simulink model "simulation_w_switch"  (Simulink 10.0)
settings: Solver=VariableStepAuto  StartTime=0.0  StopTime=tTot  MaxStep=1e-4  RelTol=1e-3
PreLoadFcn:
  | syst_init
values from neighbouring files (symbols this model uses):
  D = diag(Ir.^-1)    [syst_init.m]
  DGU = stateDyn(DGU,6)    [syst_init.m]
  Il_bar1 = 5/3    (= 1.66666666667)    [syst_init.m]
  Il_bar2 = 6/3    (= 2)    [syst_init.m]
  Il_bar3 = 7/3    (= 2.33333333333)    [syst_init.m]
  Il_bar4 = 6.5/3    (= 2.16666666667)    [syst_init.m]
  Il_bar5 = 8/3    (= 2.66666666667)    [syst_init.m]
  Il_bar6 = 7.5/3    (= 2.5)    [syst_init.m]
  L_first = Bc_first*Wcomm_first*(Bc_first')    [syst_init.m]
  L_full = Bc_full*Wcomm_full*(Bc_full')    [syst_init.m]
  L_unp = Bc_unp*Wcomm_unp*(Bc_unp')    [syst_init.m]
  N = 6    [syst_init.m]
  Pl_bar1 = 100/3    (= 33.3333333333)    [syst_init.m]
  Pl_bar2 = 120/3    (= 40)    [syst_init.m]
  Pl_bar3 = 105/3    (= 35)    [syst_init.m]
  Pl_bar4 = 95/3    (= 31.6666666667)    [syst_init.m]
  Pl_bar5 = 110/3    (= 36.6666666667)    [syst_init.m]
  Pl_bar6 = 105/3    (= 35)    [syst_init.m]
  T_zie_change = 17    [syst_init.m]
  T_zip_change = 6    [syst_init.m]
  Tc = 1.5    [syst_init.m]
  Tcommfail = tTot-3    (= 26)    [syst_init.m]
  Tplg = 10    [syst_init.m]
  Tunp = 22    [syst_init.m]
  Vref1 = 47    [syst_init.m]
  Vref2 = 48    [syst_init.m]
  Vref3 = 45    [syst_init.m]
  Vref4 = 50    [syst_init.m]
  Vref5 = 46    [syst_init.m]
  Vref6 = 49    [syst_init.m]
  Vs = 80    [syst_init.m]
  Yl_bar1 = 1/10/3    (= 0.0333333333333)    [syst_init.m]
  Yl_bar2 = 1/9/3    (= 0.037037037037)    [syst_init.m]
  Yl_bar3 = 1/11/3    (= 0.030303030303)    [syst_init.m]
  Yl_bar4 = 1/11/3    (= 0.030303030303)    [syst_init.m]
  Yl_bar5 = 1/10/3    (= 0.0333333333333)    [syst_init.m]
  Yl_bar6 = 1/10.5/3    (= 0.031746031746)    [syst_init.m]
undefined symbols (not defined in the file or in its folder): L
libraries: powerlib x135, powerlib_meascontrol x6
(part 1 of 2)
settings Model: Creator=mustafa  LastModifiedBy=mustafa
settings DataIOCC: SaveFormat=Dataset
settings OptimizationCC: LifeSpan=auto
settings DebuggingCC: UnderspecifiedInitializationDetection=Simplified  MergeDetectMultiDrivingBlocksExec=error  UnconnectedInputMsg=none  UnconnectedOutputMsg=none  UnconnectedLineMsg=none  SFUnexpectedBacktrackingDiag=error  SFNoUnconditionalDefaultTransitionDiag=error  SFExecutionAtInitializationDiag=warning
settings HardwareCC: ProdBitPerPointer=64  ProdBitPerSizeT=64  ProdBitPerPtrDiffT=64  ProdLargestAtomicFloat=Float  ProdIntDivRoundTo=Zero  ProdEndianess=LittleEndian  ProdWordSize=64  ProdHWDeviceType=Intel->x86-64 (Windows64)
settings ModelReferenceCC: PropagateSignalLabelsOutOfModel=on
settings SFSimCC: SimUseLocalCustomCode=on
settings RTWCC: RTWUseLocalCustomCode=on
settings CodeAppCC: StateflowObjectComments=off
settings GRTTargetCC: TargetLangStandard=C99 (ISO)  CombineOutputUpdateFcns=on  GRTInterface=off
settings ConfigComp: CovMetricSettings=dwe  CovHtmlReporting=off  CovSaveCumulativeToWorkspaceVar=off  CovSaveSingleToWorkspaceVar=off

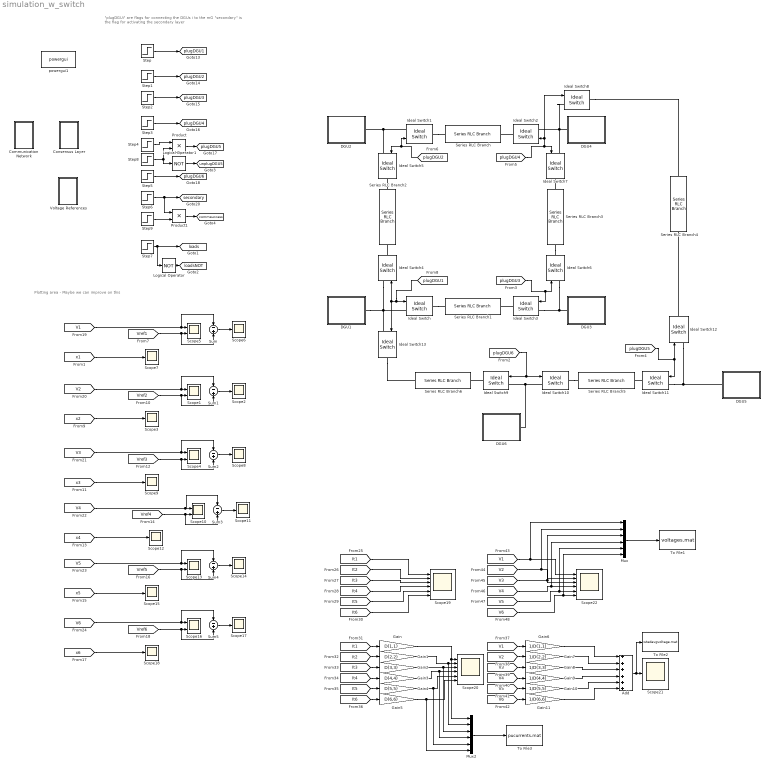
== system simulation_w_switch ==
  note: Plotting area - Maybe we can improve on this
  note: "plugDGUi" are flags for connecting the DGUs i to the mG
      | "secondary" is the flag for activating the secondary layer
  Add : Sum  Inputs=++++++
  Communication  Network : Subsystem
  Consensus Layer : Subsystem
  DGU1 : Subsystem
  DGU2 : Subsystem
  DGU3 : Subsystem
  DGU4 : Subsystem
  DGU5 : Subsystem
  DGU6 : Subsystem
  Gain : Gain  Gain=D(1,1)
  Gain1 : Gain  Gain=D(2,2)
  Gain10 : Gain  Gain=1/D(5,5)
  Gain11 : Gain  Gain=1/D(6,6)
  Gain2 : Gain  Gain=D(3,3)
  Gain3 : Gain  Gain=D(4,4)
  Gain4 : Gain  Gain=D(5,5)
  Gain5 : Gain  Gain=D(6,6)
  Gain6 : Gain  Gain=1/D(1,1)
  Gain7 : Gain  Gain=1/D(2,2)
  Gain8 : Gain  Gain=1/D(3,3)
  Gain9 : Gain  Gain=1/D(4,4)
  Ideal Switch{,1..13} (14 alike) : powerlib/Power Electronics/Ideal Switch  Ron=0.001  Lon=0  IC=0  Rs=1e5  Cs=inf  Measurements=off
      settings: SourceProductName=Simscape Electrical
  Logical Operator : Logic  Operator=NOT  AllPortsSameDT=off  OutDataTypeStr=boolean
  Logical Operator1 : Logic  Operator=NOT  AllPortsSameDT=off  OutDataTypeStr=boolean
  Mux : Mux  Inputs=6
  Mux2 : Mux  Inputs=6
  Product : Product
  Product1 : Product
  Scope{1,4..5,10,13,16} (6 alike) : Scope  NumInputPorts=2
  Scope{2..3,6..9,11..12,14..15,17..18,21} (13 alike) : Scope
  Scope19 : Scope  NumInputPorts=6
  Scope20 : Scope  NumInputPorts=6
  Scope22 : Scope  NumInputPorts=6
  Series RLC Branch : powerlib/Elements/Series RLC Branch  LConnTagsString=__new0  RConnTagsString=__new0  BranchType=RL  Resistance=DGU(2).Rij(2)  Inductance=DGU(2).Lij(2)  SetiL0=off  InitialCurrent=0  Capacitance=1e-6  Setx0=off  InitialVoltage=0  Measurements=None
      settings: SourceProductName=Simscape Electrical
  Series RLC Branch1 : powerlib/Elements/Series RLC Branch  LConnTagsString=__new0  RConnTagsString=__new0  BranchType=RL  Resistance=DGU(1).Rij(2)  Inductance=DGU(1).Lij(2)  SetiL0=off  InitialCurrent=0  Capacitance=1e-6  Setx0=off  InitialVoltage=0  Measurements=None
      settings: SourceProductName=Simscape Electrical
  Series RLC Branch2 : powerlib/Elements/Series RLC Branch  LConnTagsString=__new0  RConnTagsString=__new0  BranchType=RL  Resistance=DGU(1).Rij(1)  Inductance=DGU(1).Lij(1)  SetiL0=off  InitialCurrent=0  Capacitance=1e-6  Setx0=off  InitialVoltage=0  Measurements=None
      settings: SourceProductName=Simscape Electrical
  Series RLC Branch3 : powerlib/Elements/Series RLC Branch  LConnTagsString=__new0  RConnTagsString=__new0  BranchType=RL  Resistance=DGU(3).Rij(2)  Inductance=DGU(3).Lij(2)  SetiL0=off  InitialCurrent=0  Capacitance=1e-6  Setx0=off  InitialVoltage=0  Measurements=None
      settings: SourceProductName=Simscape Electrical
  Series RLC Branch4 : powerlib/Elements/Series RLC Branch  LConnTagsString=__new0  RConnTagsString=__new0  BranchType=RL  Resistance=DGU(4).Rij(3)  Inductance=DGU(4).Lij(3)  SetiL0=off  InitialCurrent=0  Capacitance=1e-6  Setx0=off  InitialVoltage=0  Measurements=None
      settings: SourceProductName=Simscape Electrical
  Series RLC Branch5 : powerlib/Elements/Series RLC Branch  LConnTagsString=__new0  RConnTagsString=__new0  BranchType=RL  Resistance=DGU(5).Rij(2)  Inductance=DGU(5).Lij(2)  SetiL0=off  InitialCurrent=0  Capacitance=1e-6  Setx0=off  InitialVoltage=0  Measurements=None
      settings: SourceProductName=Simscape Electrical
  Series RLC Branch6 : powerlib/Elements/Series RLC Branch  LConnTagsString=__new0  RConnTagsString=__new0  BranchType=RL  Resistance=DGU(1).Rij(3)  Inductance=DGU(1).Lij(3)  SetiL0=off  InitialCurrent=0  Capacitance=1e-6  Setx0=off  InitialVoltage=0  Measurements=None
      settings: SourceProductName=Simscape Electrical
  Step{,1..4,6} (6 alike) : Step  Time=Tc  SampleTime=0
  Step5 : Step  Time=Tplg  SampleTime=0
  Step7 : Step  Time=Tc-0.1  SampleTime=0
  Step8 : Step  Time=Tunp  Before=1  After=0  SampleTime=0
  Step9 : Step  Time=Tcommfail  Before=1  After=0  SampleTime=0
  Sum{,1..5} (6 alike) : Sum  Inputs=-|+
  To File1 : ToFile  Filename=voltages.mat  MatrixName=V  SaveFormat=Timeseries
  To File2 : ToFile  Filename=wtedavgvoltage.mat  MatrixName=Vavg  SaveFormat=Timeseries
  To File3 : ToFile  Filename=pucurrents.mat  MatrixName=Itpu  SaveFormat=Timeseries
  Voltage References : Subsystem
  powergui1 : powerlib/powergui  Priority=1  SimulationMode=Continuous  SampleTime=50e-6  frequency=60  Iterations=50  frequencyindice=0  Pbase=100e6  ErrMax=1e-4  UnitsV=kV  UnitsW=MW  buscounter=0  FunctionMessages=off  echomessages=off  EnableUseOfTLC=off  CurrentSourceSwitches=off  DisableSnubberDevices=off  DisableRonSwitches=off  DisableVfSwitches=off  DisplayEquations=off  AutomaticDiscreteSolvers=off  SolverType=Tustin/Backward Euler (TBE)  Interpol=off  ExternalGateDelay=off  methode=off  Ts=100  x0status=blocks  SPID=on  SwTol=0  HookPort=off  NonlinearTolerance=1e-4  nMaxIteration=100  ContinueOnMaxIteration=off  RestoreLinks=warning  ResistiveCurrentMeasurement=off  Frange=[0:2:500]  Ylog=off  Xlog=on  ShowGrid=off  save=off  variable=ZData  structure=0  ZoomFFT=off  StartTime=0.0  cycles=1  DisplayStyle=1  fundamental=60  FreqAxis=off  MaxFrequency=1000  frequencyindicesteady=1  RmsSteady=1  display=off
      settings: SourceProductName=Simscape Electrical
  tag scope: commsuccess=global, loads=global, loadsNOT=global, plugDGU1=global, plugDGU2=global, plugDGU3=global, plugDGU4=global, plugDGU5=global, plugDGU6=global, secondary=global, unplugDGU5=global
  wires:
  [Vref1] -> Sum/2, Scope5/2
  [V1] -> Sum/1, Scope5/1
  Sum/1 -> Scope6/1
  [x1] -> Scope7/1
  [plugDGU2] -> Ideal Switch1/1, Ideal Switch5/1
  [plugDGU1] -> Ideal Switch4/1, Ideal Switch13/1, Ideal Switch/1
  [plugDGU3] -> Ideal Switch6/1, Ideal Switch3/1
  [plugDGU4] -> Ideal Switch7/1, Ideal Switch8/1, Ideal Switch2/1
  [plugDGU6] -> Ideal Switch9/1, Ideal Switch10/1
  [plugDGU5] -> Ideal Switch11/1, Ideal Switch12/1
  [V2] -> Sum1/1, Scope1/1
  [Vref2] -> Sum1/2, Scope1/2
  Sum1/1 -> Scope2/1
  [x2] -> Scope3/1
  [V3] -> Sum2/1, Scope4/1
  [Vref3] -> Sum2/2, Scope4/2
  Sum2/1 -> Scope8/1
  [x3] -> Scope9/1
  [V4] -> Sum3/1, Scope10/1
  [Vref4] -> Sum3/2, Scope10/2
  Sum3/1 -> Scope11/1
  [x4] -> Scope12/1
  [V5] -> Sum4/1, Scope13/1
  [Vref5] -> Sum4/2, Scope13/2
  Sum4/1 -> Scope14/1
  [x5] -> Scope15/1
  [V6] -> Sum5/1, Scope16/1
  [Vref6] -> Sum5/2, Scope16/2
  Sum5/1 -> Scope17/1
  [x6] -> Scope18/1
  Step/1 -> [plugDGU1]
  Step1/1 -> [plugDGU2]
  Step2/1 -> [plugDGU3]
  Step3/1 -> [plugDGU4]
  Step5/1 -> [plugDGU6]
  Step6/1 -> Product1/1, [secondary]
  [It3] -> Scope19/3
  [It2] -> Scope19/2
  [It1] -> Scope19/1
  [It4] -> Scope19/4
  [It5] -> Scope19/5
  [It6] -> Scope19/6
  [V6] -> Mux/6, Scope22/6
  [V1] -> Mux/1, Scope22/1
  [V4] -> Mux/4, Scope22/4
  [V3] -> Mux/3, Scope22/3
  [V2] -> Mux/2, Scope22/2
  [V5] -> Mux/5, Scope22/5
  Step7/1 -> Logical Operator/1, [loads]
  Logical Operator/1 -> [loadsNOT]
  Product/1 -> [plugDGU5]
  Step4/1 -> Product/1
  Step8/1 -> Logical Operator1/1, Product/2
  Logical Operator1/1 -> [unplugDGU5]
  [It1] -> Gain/1
  [It2] -> Gain1/1
  [It3] -> Gain2/1
  [It4] -> Gain3/1
  [It5] -> Gain4/1
  [It6] -> Gain5/1
  Gain5/1 -> Mux2/6, Scope20/6
  Gain4/1 -> Mux2/5, Scope20/5
  Gain3/1 -> Mux2/4, Scope20/4
  Gain2/1 -> Scope20/3, Mux2/3
  Gain1/1 -> Mux2/2, Scope20/2
  Gain/1 -> Mux2/1, Scope20/1
  Step9/1 -> Product1/2
  Product1/1 -> [commsuccess]
  Gain6/1 -> Add/1
  Gain7/1 -> Add/2
  Gain8/1 -> Add/3
  Gain9/1 -> Add/4
  Gain10/1 -> Add/5
  Gain11/1 -> Add/6
  [V6] -> Gain11/1
  [V5] -> Gain10/1
  [V4] -> Gain9/1
  [V3] -> Gain8/1
  [V2] -> Gain7/1
  [V1] -> Gain6/1
  Mux/1 -> To File1/1
  Mux2/1 -> To File3/1
  Add/1 -> To File2/1, Scope21/1
  connections:
  Ideal Switch/RConn1 -- Series RLC Branch1/LConn1
  Ideal Switch1/RConn1 -- Series RLC Branch/LConn1
  Ideal Switch4/RConn1 -- Series RLC Branch2/RConn1
  DGU1/RConn1 -- Ideal Switch13/LConn1 -- Ideal Switch4/LConn1 -- Ideal Switch/LConn1
  Ideal Switch5/RConn1 -- Series RLC Branch2/LConn1
  Ideal Switch1/LConn1 -- Ideal Switch5/LConn1 -- DGU2/RConn1
  Ideal Switch3/RConn1 -- Series RLC Branch1/RConn1
  Ideal Switch2/RConn1 -- Series RLC Branch/RConn1
  Ideal Switch3/LConn1 -- Ideal Switch6/LConn1 -- DGU3/LConn1
  Ideal Switch2/LConn1 -- Ideal Switch8/LConn1 -- Ideal Switch7/LConn1 -- DGU4/LConn1
  Series RLC Branch3/LConn1 -- Ideal Switch7/RConn1
  Series RLC Branch3/RConn1 -- Ideal Switch6/RConn1
  Ideal Switch8/RConn1 -- Series RLC Branch4/LConn1
  Ideal Switch9/RConn1 -- Series RLC Branch6/RConn1
  Ideal Switch10/RConn1 -- Series RLC Branch5/LConn1
  Ideal Switch10/LConn1 -- Ideal Switch9/LConn1 -- DGU6/RConn1
  Ideal Switch11/RConn1 -- Series RLC Branch5/RConn1
  Ideal Switch11/LConn1 -- Ideal Switch12/LConn1 -- DGU5/LConn1
  Ideal Switch13/RConn1 -- Series RLC Branch6/LConn1
  Ideal Switch12/RConn1 -- Series RLC Branch4/RConn1

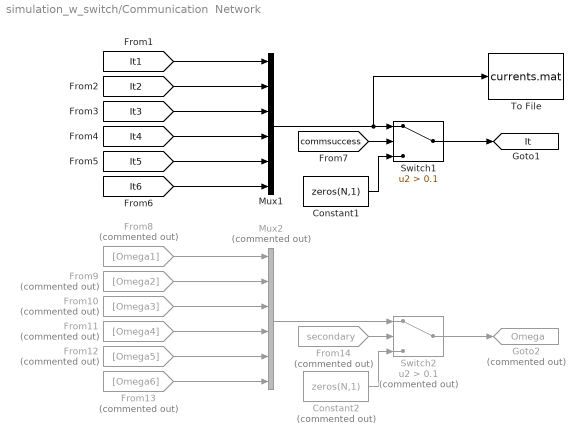
== system simulation_w_switch/Communication  Network ==
  Constant1 : Constant  Value=zeros(N,1)
  Constant2 : Constant  Commented=on  Value=zeros(N,1)
  From10 : From  Commented=on  GotoTag=Omega3  TagVisibility=global
  From11 : From  Commented=on  GotoTag=Omega4  TagVisibility=global
  From12 : From  Commented=on  GotoTag=Omega5  TagVisibility=global
  From13 : From  Commented=on  GotoTag=Omega6  TagVisibility=global
  From14 : From  Commented=on  GotoTag=secondary  TagVisibility=global
  From8 : From  Commented=on  GotoTag=Omega1  TagVisibility=global
  From9 : From  Commented=on  GotoTag=Omega2  TagVisibility=global
  Goto2 : Goto  Commented=on  GotoTag=Omega  TagVisibility=global
  Mux1 : Mux  Inputs=6
  Mux2 : Mux  Commented=on  Inputs=6
  Switch1 : Switch  Criteria=u2 > Threshold  Threshold=0.1
  Switch2 : Switch  Commented=on  Criteria=u2 > Threshold  Threshold=0.1
  To File : ToFile  Filename=currents.mat  MatrixName=It  SaveFormat=Timeseries
  tag scope: It=global
  wires:
  Mux1/1 -> To File/1, Switch1/1
  Switch1/1 -> [It]
  [commsuccess] -> Switch1/2
  Constant1/1 -> Switch1/3
  [It2] -> Mux1/2
  [It3] -> Mux1/3
  [It4] -> Mux1/4
  [It5] -> Mux1/5
  [It6] -> Mux1/6
  [It1] -> Mux1/1
  From8/1 -> Mux2/1
  From13/1 -> Mux2/6
  From12/1 -> Mux2/5
  From11/1 -> Mux2/4
  From10/1 -> Mux2/3
  From9/1 -> Mux2/2
  Constant2/1 -> Switch2/3
  From14/1 -> Switch2/2
  Switch2/1 -> Goto2/1
  Mux2/1 -> Switch2/1

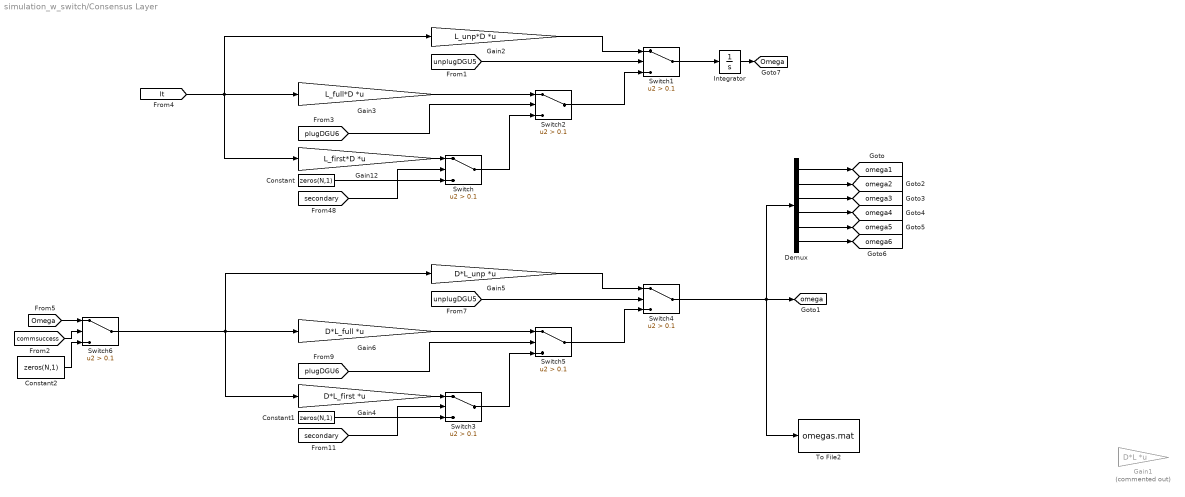
== system simulation_w_switch/Consensus Layer ==
  Constant : Constant  Value=zeros(N,1)
  Constant1 : Constant  Value=zeros(N,1)
  Constant2 : Constant  Value=zeros(N,1)
  Demux : Demux  Outputs=6
  Gain1 : Gain  Commented=on  Gain=D*L  Multiplication=Matrix(K*u) (u vector)
  Gain12 : Gain  Gain=L_first*D  Multiplication=Matrix(K*u) (u vector)
  Gain2 : Gain  Gain=L_unp*D  Multiplication=Matrix(K*u) (u vector)
  Gain3 : Gain  Gain=L_full*D  Multiplication=Matrix(K*u) (u vector)
  Gain4 : Gain  Gain=D*L_first  Multiplication=Matrix(K*u) (u vector)
  Gain5 : Gain  Gain=D*L_unp  Multiplication=Matrix(K*u) (u vector)
  Gain6 : Gain  Gain=D*L_full  Multiplication=Matrix(K*u) (u vector)
  Integrator : Integrator
  Switch{,1..6} (7 alike) : Switch  Criteria=u2 > Threshold  Threshold=0.1
  To File2 : ToFile  Filename=omegas.mat  MatrixName=omega  SaveFormat=Timeseries
  tag scope: Omega=global, omega1=global, omega2=global, omega3=global, omega4=global, omega5=global, omega6=global, omega=global
  wires:
  Constant/1 -> Switch/3
  [secondary] -> Switch/2
  Switch4/1 -> To File2/1, Demux/1, [omega]
  Gain12/1 -> Switch/1
  Demux/1 -> [omega1]
  Demux/6 -> [omega6]
  Demux/5 -> [omega5]
  Demux/4 -> [omega4]
  Demux/3 -> [omega3]
  Demux/2 -> [omega2]
  Switch1/1 -> Integrator/1
  Switch2/1 -> Switch1/3
  [unplugDGU5] -> Switch1/2
  Gain2/1 -> Switch1/1
  [It] -> Gain12/1, Gain2/1, Gain3/1
  Switch/1 -> Switch2/3
  [plugDGU6] -> Switch2/2
  Gain3/1 -> Switch2/1
  Integrator/1 -> [Omega]
  Gain6/1 -> Switch5/1
  [plugDGU6] -> Switch5/2
  Switch3/1 -> Switch5/3
  Gain5/1 -> Switch4/1
  [unplugDGU5] -> Switch4/2
  Switch5/1 -> Switch4/3
  Gain4/1 -> Switch3/1
  [secondary] -> Switch3/2
  Constant1/1 -> Switch3/3
  Switch6/1 -> Gain4/1, Gain6/1, Gain5/1
  Constant2/1 -> Switch6/3
  [commsuccess] -> Switch6/2
  [Omega] -> Switch6/1

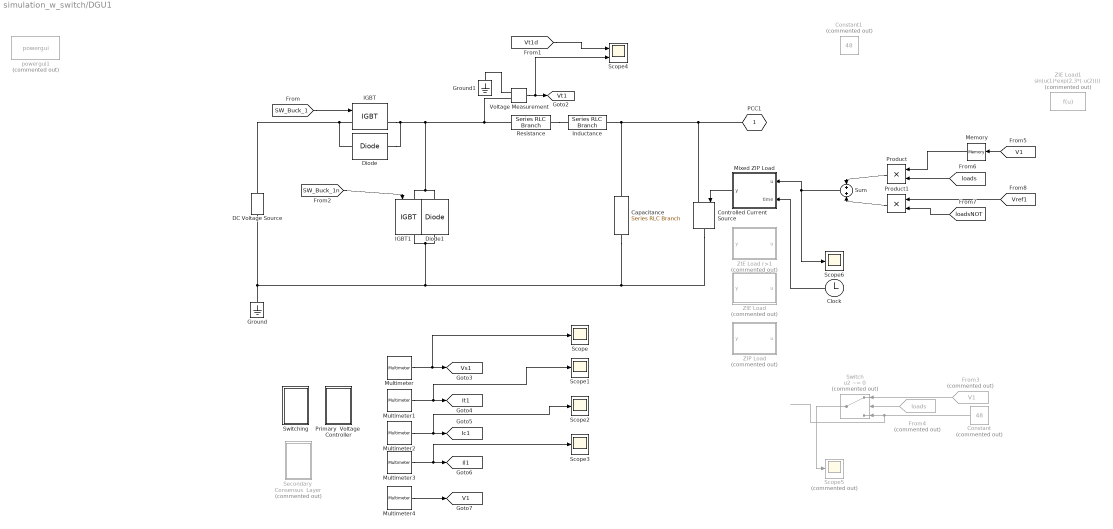
== system simulation_w_switch/DGU1 ==
  Capacitance : powerlib/Elements/Series RLC Branch  LConnTagsString=__new0  RConnTagsString=__new0  BranchType=C  Resistance=1  Inductance=1.8e-3  SetiL0=off  InitialCurrent=0  Capacitance=DGU(1).Ct  Setx0=on  InitialVoltage=48  Measurements=Branch voltage and current
      settings: SourceProductName=Simscape Electrical
  Clock : Clock
  Constant : Constant  Commented=on  Value=48
  Constant1 : Constant  Commented=on  Value=48
  Controlled Current Source : powerlib/Electrical Sources/Controlled Current Source  Initialize=on  Source_Type=DC  Amplitude=Il_bar1  Phase=0  Frequency=0  Measurements=Current
      settings: SourceProductName=Simscape Electrical
  DC Voltage Source : powerlib/Electrical Sources/DC Voltage Source  Amplitude=Vs  Measurements=Voltage
      settings: SourceProductName=Simscape Electrical
  Diode : powerlib/Power Electronics/Diode  Ron=0.001  Lon=0  Vf=0.8  IC=0  UseSnubber=0  Rs=500  Cs=250e-9  Measurements=off
      settings: SourceProductName=Simscape Electrical
  Diode1 : powerlib/Power Electronics/Diode  Ron=0.001  Lon=0  Vf=0.8  IC=0  UseSnubber=0  Rs=500  Cs=250e-9  Measurements=off
      settings: SourceProductName=Simscape Electrical
  From3 : From  Commented=on  GotoTag=V1  TagVisibility=global
  From4 : From  Commented=on  GotoTag=loads  TagVisibility=global
  Ground : powerlib/Elements/Ground  LConnTagsString=a
      settings: SourceProductName=Simscape Electrical
  Ground1 : powerlib/Elements/Ground  LConnTagsString=a
      settings: SourceProductName=Simscape Electrical
  IGBT : powerlib/Power Electronics/IGBT  Ron=0.001  Lon=0  Vf=1  Tf=1e-6  Tt=2e-6  IC=0  Rs=1e5  Cs=inf  Measurements=on
      settings: SourceProductName=Simscape Electrical
  IGBT1 : powerlib/Power Electronics/IGBT  Ron=0.001  Lon=0  Vf=1  Tf=1e-6  Tt=2e-6  IC=0  Rs=1e5  Cs=inf  Measurements=on
      settings: SourceProductName=Simscape Electrical
  Inductance : powerlib/Elements/Series RLC Branch  LConnTagsString=__new0  RConnTagsString=__new0  BranchType=L  Resistance=1  Inductance=DGU(1).Lt  SetiL0=on  InitialCurrent=Il_bar1  Capacitance=1e-6  Setx0=off  InitialVoltage=0  Measurements=None
      settings: SourceProductName=Simscape Electrical
  Memory : Memory
  Mixed ZIP Load : MATLAB Function  TreatAsAtomicUnit=on
  Multimeter : powerlib/Measurements/Multimeter  PhasorSimulation=off  OutputType=Complex  sel=7  L=30  Gain=1  yselected={'Usrc: DGU1/DC Voltage Source'};  PSBOutputType=1  PSBequivalent=0  AxesSetting=[0,0.1,-100,100]  Display=0  SavedBlockNames=-11
      settings: SourceProductName=Simscape Electrical
  Multimeter1 : powerlib/Measurements/Multimeter  PhasorSimulation=off  OutputType=Complex  sel=14  L=30  Gain=1  yselected={'Ib: DGU1/Resistance'};  PSBOutputType=1  PSBequivalent=0  AxesSetting=[0,0.1,-100,100]  Display=0  SavedBlockNames=-11
      settings: SourceProductName=Simscape Electrical
  Multimeter2 : powerlib/Measurements/Multimeter  PhasorSimulation=off  OutputType=Complex  sel=13  L=30  Gain=1  yselected={'Ib: DGU1/Capacitance'};  PSBOutputType=1  PSBequivalent=0  AxesSetting=[0,0.1,-100,100]  Display=0  SavedBlockNames=-11
      settings: SourceProductName=Simscape Electrical
  Multimeter3 : powerlib/Measurements/Multimeter  PhasorSimulation=off  OutputType=Complex  sel=25  L=30  Gain=1  yselected={'Isrc: DGU1/Controlled Current Source'};  PSBOutputType=1  PSBequivalent=0  AxesSetting=[0,0.1,-100,100]  Display=0  SavedBlockNames=-11
      settings: SourceProductName=Simscape Electrical
  Multimeter4 : powerlib/Measurements/Multimeter  PhasorSimulation=off  OutputType=Complex  sel=1  L=30  Gain=1  yselected={'Ub: DGU1/Capacitance'};  PSBOutputType=1  PSBequivalent=0  AxesSetting=[0,0.1,-100,100]  Display=0  SavedBlockNames=-11
      settings: SourceProductName=Simscape Electrical
  Primary  Voltage  Controller : Subsystem
  Product : Product
  Product1 : Product
  Resistance : powerlib/Elements/Series RLC Branch  LConnTagsString=__new0  RConnTagsString=__new0  BranchType=R  Resistance=DGU(1).Rt  Inductance=1e-3  SetiL0=off  InitialCurrent=0  Capacitance=1e-6  Setx0=off  InitialVoltage=0  Measurements=Branch current
      settings: SourceProductName=Simscape Electrical
  Scope{,1..3,6} (5 alike) : Scope
  Scope4 : Scope  NumInputPorts=2
  Scope5 : Scope  Commented=on
  Secondary  Consensus  Layer : Subsystem  Commented=on
  Sum : Sum  Inputs=+|+
  Switch : Switch  Commented=on  Criteria=u2 ~= 0  Threshold=0.1
  Switching : Subsystem
  Voltage Measurement : powerlib/Measurements/Voltage Measurement  PhasorSimulation=off  OutputType=Complex  PSBequivalent=0
      settings: SourceProductName=Simscape Electrical
  ZIE Load : MATLAB Function  Commented=on  TreatAsAtomicUnit=on
  ZIE Load r>1 : MATLAB Function  Commented=on  TreatAsAtomicUnit=on
  ZIE Load1 : Fcn  Commented=on  Expr=sin(u(1)*exp(2.3*(-u(2))))
  ZIP Load : MATLAB Function  Commented=on  TreatAsAtomicUnit=on
  powergui1 : powerlib/powergui  Priority=1  Commented=on  SimulationMode=Continuous  SampleTime=50e-6  frequency=60  Iterations=50  frequencyindice=60  Pbase=100e6  ErrMax=1e-4  UnitsV=kV  UnitsW=MW  buscounter=0  FunctionMessages=off  echomessages=off  EnableUseOfTLC=off  CurrentSourceSwitches=off  DisableSnubberDevices=off  DisableRonSwitches=off  DisableVfSwitches=off  DisplayEquations=off  AutomaticDiscreteSolvers=off  SolverType=Tustin/Backward Euler (TBE)  Interpol=off  ExternalGateDelay=off  methode=off  Ts=100  x0status=blocks  SPID=on  SwTol=0  HookPort=off  NonlinearTolerance=1e-4  nMaxIteration=100  ContinueOnMaxIteration=off  RestoreLinks=warning  ResistiveCurrentMeasurement=off  Frange=[0:2:500]  Ylog=off  Xlog=on  ShowGrid=off  save=off  variable=ZData  structure=0  ZoomFFT=off  StartTime=0.0  cycles=1  DisplayStyle=1  fundamental=60  FreqAxis=off  MaxFrequency=1000  frequencyindicesteady=1  RmsSteady=1  display=off
      settings: SourceProductName=Simscape Electrical
  PCC1 : PMIOPort  Tag=PMCPort  Side=Right
  tag scope: Ic1=global, Il1=global, It1=global, V1=global, Vs1=global, Vt1=global
  wires:
  Multimeter/1 -> Scope/1, [Vs1]
  Multimeter2/1 -> Scope2/1, [Ic1]
  Voltage Measurement/1 -> Scope4/2, [Vt1]
  Multimeter1/1 -> Scope1/1, [It1]
  [SW_Buck_1n] -> IGBT1/1
  Multimeter3/1 -> Scope3/1, [Il1]
  [SW_Buck_1] -> IGBT/1
  Multimeter4/1 -> [V1]
  [Vt1d] -> Scope4/1
  Mixed ZIP Load/1(y) -> Controlled Current Source/1
  From4/1 -> Switch/2
  From3/1 -> Switch/1
  Constant/1 -> Switch/3
  Switch/1 -> Scope5/1
  [loads] -> Product/2
  [Vref1] -> Product1/1
  [loadsNOT] -> Product1/2
  Product/1 -> Sum/1
  Product1/1 -> Sum/2
  Sum/1 -> Mixed ZIP Load/1(u), Scope6/1
  [V1] -> Memory/1
  Memory/1 -> Product/1
  Clock/1 -> Mixed ZIP Load/2(time)
  connections:
  Ground1/LConn1 -- Voltage Measurement/LConn2
  IGBT1/RConn1 -- Controlled Current Source/RConn1 -- Capacitance/RConn1 -- Ground/LConn1 -- DC Voltage Source/LConn1 -- Diode1/LConn1
  Capacitance/LConn1 -- Controlled Current Source/LConn1 -- PCC1/RConn1 -- Inductance/RConn1
  IGBT1/LConn1 -- Resistance/LConn1 -- Voltage Measurement/LConn1 -- IGBT/RConn1 -- Diode/LConn1 -- Diode1/RConn1
  IGBT/LConn1 -- Diode/RConn1 -- DC Voltage Source/RConn1
  Resistance/RConn1 -- Inductance/LConn1

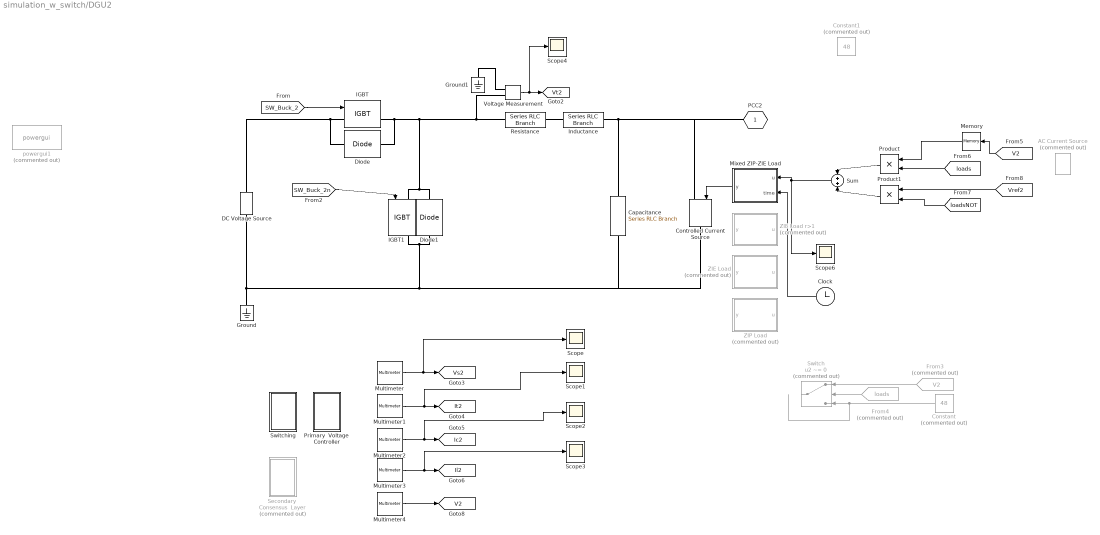
== system simulation_w_switch/DGU2 ==
  AC Current Source : powerlib/Electrical Sources/AC Current Source  Commented=on  Amplitude=12  Phase=90  Frequency=0  SampleTime=0  Measurements=Current
      settings: SourceProductName=Simscape Electrical  SourceProductBaseCode=PS
  Capacitance : powerlib/Elements/Series RLC Branch  LConnTagsString=__new0  RConnTagsString=__new0  BranchType=C  Resistance=1  Inductance=1.8e-3  SetiL0=off  InitialCurrent=0  Capacitance=DGU(2).Ct  Setx0=on  InitialVoltage=48  Measurements=Branch voltage and current
      settings: SourceProductName=Simscape Electrical
  Clock : Clock
  Constant : Constant  Commented=on  Value=48
  Constant1 : Constant  Commented=on  Value=48
  Controlled Current Source : powerlib/Electrical Sources/Controlled Current Source  Initialize=on  Source_Type=DC  Amplitude=Il_bar2  Phase=0  Frequency=0  Measurements=Current
      settings: SourceProductName=Simscape Electrical
  DC Voltage Source : powerlib/Electrical Sources/DC Voltage Source  Amplitude=Vs  Measurements=Voltage
      settings: SourceProductName=Simscape Electrical
  Diode : powerlib/Power Electronics/Diode  Ron=0.001  Lon=0  Vf=0.8  IC=0  UseSnubber=0  Rs=500  Cs=250e-9  Measurements=off
      settings: SourceProductName=Simscape Electrical
  Diode1 : powerlib/Power Electronics/Diode  Ron=0.001  Lon=0  Vf=0.8  IC=0  UseSnubber=0  Rs=500  Cs=250e-9  Measurements=off
      settings: SourceProductName=Simscape Electrical
  From3 : From  Commented=on  GotoTag=V2  TagVisibility=global
  From4 : From  Commented=on  GotoTag=loads  TagVisibility=global
  Ground : powerlib/Elements/Ground  LConnTagsString=a
      settings: SourceProductName=Simscape Electrical
  Ground1 : powerlib/Elements/Ground  LConnTagsString=a
      settings: SourceProductName=Simscape Electrical
  IGBT : powerlib/Power Electronics/IGBT  Ron=0.001  Lon=0  Vf=1  Tf=1e-6  Tt=2e-6  IC=0  Rs=1e5  Cs=inf  Measurements=on
      settings: SourceProductName=Simscape Electrical
  IGBT1 : powerlib/Power Electronics/IGBT  Ron=0.001  Lon=0  Vf=1  Tf=1e-6  Tt=2e-6  IC=0  Rs=1e5  Cs=inf  Measurements=on
      settings: SourceProductName=Simscape Electrical
  Inductance : powerlib/Elements/Series RLC Branch  LConnTagsString=__new0  RConnTagsString=__new0  BranchType=L  Resistance=1  Inductance=DGU(2).Lt  SetiL0=on  InitialCurrent=Il_bar2  Capacitance=1e-6  Setx0=off  InitialVoltage=0  Measurements=None
      settings: SourceProductName=Simscape Electrical
  Memory : Memory
  Mixed ZIP-ZIE Load : MATLAB Function  TreatAsAtomicUnit=on
  Multimeter : powerlib/Measurements/Multimeter  PhasorSimulation=off  OutputType=Complex  sel=8  L=30  Gain=1  yselected={'Usrc: DGU2/DC Voltage Source'};  PSBOutputType=1  PSBequivalent=0  AxesSetting=[0,0.1,-100,100]  Display=0  SavedBlockNames=-11
      settings: SourceProductName=Simscape Electrical
  Multimeter1 : powerlib/Measurements/Multimeter  PhasorSimulation=off  OutputType=Complex  sel=16  L=30  Gain=1  yselected={'Ib: DGU2/Resistance'};  PSBOutputType=1  PSBequivalent=0  AxesSetting=[0,0.1,-100,100]  Display=0  SavedBlockNames=-11
      settings: SourceProductName=Simscape Electrical
  Multimeter2 : powerlib/Measurements/Multimeter  PhasorSimulation=off  OutputType=Complex  sel=15  L=30  Gain=1  yselected={'Ib: DGU2/Capacitance'};  PSBOutputType=1  PSBequivalent=0  AxesSetting=[0,0.1,-100,100]  Display=0  SavedBlockNames=-11
      settings: SourceProductName=Simscape Electrical
  Multimeter3 : powerlib/Measurements/Multimeter  PhasorSimulation=off  OutputType=Complex  sel=26  L=30  Gain=1  yselected={'Isrc: DGU2/Controlled Current Source'};  PSBOutputType=1  PSBequivalent=0  AxesSetting=[0,0.1,-100,100]  Display=0  SavedBlockNames=-11
      settings: SourceProductName=Simscape Electrical
  Multimeter4 : powerlib/Measurements/Multimeter  PhasorSimulation=off  OutputType=Complex  sel=2  L=30  Gain=1  yselected={'Ub: DGU2/Capacitance'};  PSBOutputType=1  PSBequivalent=0  AxesSetting=[0,0.1,-100,100]  Display=0  SavedBlockNames=-11
      settings: SourceProductName=Simscape Electrical
  Primary  Voltage  Controller : Subsystem
  Product : Product
  Product1 : Product
  Resistance : powerlib/Elements/Series RLC Branch  LConnTagsString=__new0  RConnTagsString=__new0  BranchType=R  Resistance=DGU(2).Rt  Inductance=1e-3  SetiL0=off  InitialCurrent=0  Capacitance=1e-6  Setx0=off  InitialVoltage=0  Measurements=Branch current
      settings: SourceProductName=Simscape Electrical
  Scope{,1..4,6} (6 alike) : Scope
  Secondary  Consensus  Layer : Subsystem  Commented=on
  Sum : Sum  Inputs=+|+
  Switch : Switch  Commented=on  Criteria=u2 ~= 0  Threshold=0.1
  Switching : Subsystem
  Voltage Measurement : powerlib/Measurements/Voltage Measurement  PhasorSimulation=off  OutputType=Complex  PSBequivalent=0
      settings: SourceProductName=Simscape Electrical
  ZIE Load : MATLAB Function  Commented=on  TreatAsAtomicUnit=on
  ZIE Load r>1 : MATLAB Function  Commented=on  TreatAsAtomicUnit=on
  ZIP Load : MATLAB Function  Commented=on  TreatAsAtomicUnit=on
  powergui1 : powerlib/powergui  Priority=1  Commented=on  SimulationMode=Continuous  SampleTime=50e-6  frequency=60  Iterations=50  frequencyindice=60  Pbase=100e6  ErrMax=1e-4  UnitsV=kV  UnitsW=MW  buscounter=0  FunctionMessages=off  echomessages=off  EnableUseOfTLC=off  CurrentSourceSwitches=off  DisableSnubberDevices=off  DisableRonSwitches=off  DisableVfSwitches=off  DisplayEquations=off  AutomaticDiscreteSolvers=off  SolverType=Tustin/Backward Euler (TBE)  Interpol=off  ExternalGateDelay=off  methode=off  Ts=100  x0status=blocks  SPID=on  SwTol=0  HookPort=off  NonlinearTolerance=1e-4  nMaxIteration=100  ContinueOnMaxIteration=off  RestoreLinks=warning  ResistiveCurrentMeasurement=off  Frange=[0:2:500]  Ylog=off  Xlog=on  ShowGrid=off  save=off  variable=ZData  structure=0  ZoomFFT=off  StartTime=0.0  cycles=1  DisplayStyle=1  fundamental=60  FreqAxis=off  MaxFrequency=1000  frequencyindicesteady=1  RmsSteady=1  display=off
      settings: SourceProductName=Simscape Electrical
  PCC2 : PMIOPort  Tag=PMCPort  Side=Right
  tag scope: Ic2=global, Il2=global, It2=global, V2=global, Vs2=global, Vt2=global
  wires:
  Multimeter/1 -> Scope/1, [Vs2]
  Multimeter2/1 -> Scope2/1, [Ic2]
  Voltage Measurement/1 -> Scope4/1, [Vt2]
  Multimeter1/1 -> Scope1/1, [It2]
  [SW_Buck_2n] -> IGBT1/1
  Multimeter3/1 -> Scope3/1, [Il2]
  [SW_Buck_2] -> IGBT/1
  Multimeter4/1 -> [V2]
  Mixed ZIP-ZIE Load/1(y) -> Controlled Current Source/1
  From4/1 -> Switch/2
  From3/1 -> Switch/1
  Constant/1 -> Switch/3
  [Vref2] -> Product1/1
  Product1/1 -> Sum/2
  Sum/1 -> Mixed ZIP-ZIE Load/1(u), Scope6/1
  [loadsNOT] -> Product1/2
  [loads] -> Product/2
  Memory/1 -> Product/1
  Product/1 -> Sum/1
  [V2] -> Memory/1
  Clock/1 -> Mixed ZIP-ZIE Load/2(time)
  connections:
  Ground1/LConn1 -- Voltage Measurement/LConn2
  IGBT1/RConn1 -- Controlled Current Source/RConn1 -- Capacitance/RConn1 -- Ground/LConn1 -- DC Voltage Source/LConn1 -- Diode1/LConn1
  Diode/LConn1 -- IGBT/RConn1 -- Resistance/LConn1 -- Voltage Measurement/LConn1 -- IGBT1/LConn1 -- Diode1/RConn1
  IGBT/LConn1 -- Diode/RConn1 -- DC Voltage Source/RConn1
  Resistance/RConn1 -- Inductance/LConn1
  Capacitance/LConn1 -- PCC2/RConn1 -- Controlled Current Source/LConn1 -- Inductance/RConn1

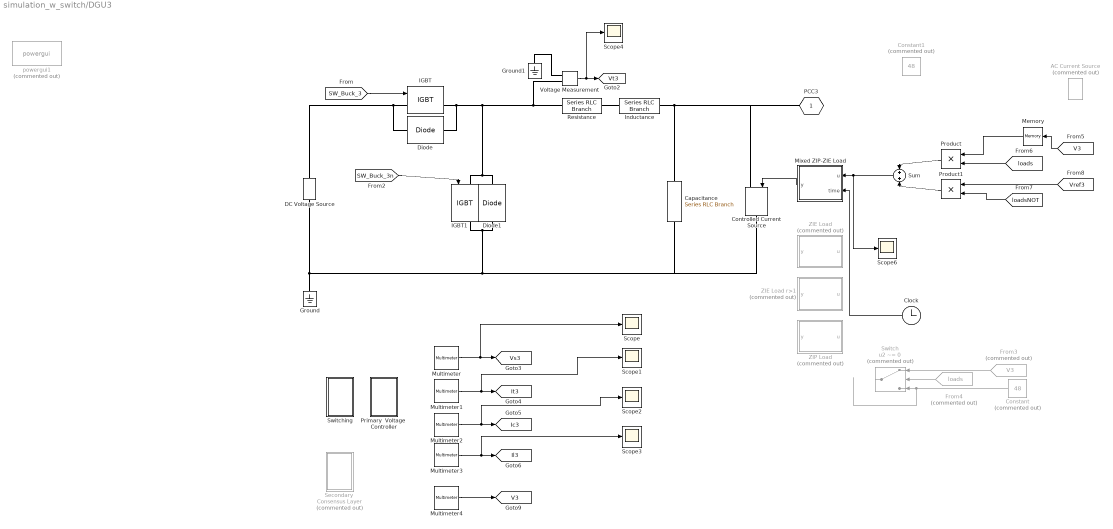
== system simulation_w_switch/DGU3 ==
  AC Current Source : powerlib/Electrical Sources/AC Current Source  Commented=on  Amplitude=15  Phase=90  Frequency=0  SampleTime=0  Measurements=Current
      settings: SourceProductName=Simscape Electrical  SourceProductBaseCode=PS
  Capacitance : powerlib/Elements/Series RLC Branch  LConnTagsString=__new0  RConnTagsString=__new0  BranchType=C  Resistance=1  Inductance=1.8e-3  SetiL0=off  InitialCurrent=0  Capacitance=DGU(3).Ct  Setx0=on  InitialVoltage=48  Measurements=Branch voltage and current
      settings: SourceProductName=Simscape Electrical
  Clock : Clock
  Constant : Constant  Commented=on  Value=48
  Constant1 : Constant  Commented=on  Value=48
  Controlled Current Source : powerlib/Electrical Sources/Controlled Current Source  Initialize=on  Source_Type=DC  Amplitude=Il_bar3  Phase=0  Frequency=0  Measurements=Current
      settings: SourceProductName=Simscape Electrical
  DC Voltage Source : powerlib/Electrical Sources/DC Voltage Source  Amplitude=Vs  Measurements=Voltage
      settings: SourceProductName=Simscape Electrical
  Diode : powerlib/Power Electronics/Diode  Ron=0.001  Lon=0  Vf=0.8  IC=0  UseSnubber=0  Rs=500  Cs=250e-9  Measurements=off
      settings: SourceProductName=Simscape Electrical
  Diode1 : powerlib/Power Electronics/Diode  Ron=0.001  Lon=0  Vf=0.8  IC=0  UseSnubber=0  Rs=500  Cs=250e-9  Measurements=off
      settings: SourceProductName=Simscape Electrical
  From3 : From  Commented=on  GotoTag=V3  TagVisibility=global
  From4 : From  Commented=on  GotoTag=loads  TagVisibility=global
  Ground : powerlib/Elements/Ground  LConnTagsString=a
      settings: SourceProductName=Simscape Electrical
  Ground1 : powerlib/Elements/Ground  LConnTagsString=a
      settings: SourceProductName=Simscape Electrical
  IGBT : powerlib/Power Electronics/IGBT  Ron=0.001  Lon=0  Vf=1  Tf=1e-6  Tt=2e-6  IC=0  Rs=1e5  Cs=inf  Measurements=on
      settings: SourceProductName=Simscape Electrical
  IGBT1 : powerlib/Power Electronics/IGBT  Ron=0.001  Lon=0  Vf=1  Tf=1e-6  Tt=2e-6  IC=0  Rs=1e5  Cs=inf  Measurements=on
      settings: SourceProductName=Simscape Electrical
  Inductance : powerlib/Elements/Series RLC Branch  LConnTagsString=__new0  RConnTagsString=__new0  BranchType=L  Resistance=1  Inductance=DGU(3).Lt  SetiL0=on  InitialCurrent=Il_bar3  Capacitance=1e-6  Setx0=off  InitialVoltage=0  Measurements=None
      settings: SourceProductName=Simscape Electrical
  Memory : Memory
  Mixed ZIP-ZIE Load : MATLAB Function  TreatAsAtomicUnit=on
  Multimeter : powerlib/Measurements/Multimeter  PhasorSimulation=off  OutputType=Complex  sel=9  L=30  Gain=1  yselected={'Usrc: DGU3/DC Voltage Source'};  PSBOutputType=1  PSBequivalent=0  AxesSetting=[0,0.1,-100,100]  Display=0  SavedBlockNames=-11
      settings: SourceProductName=Simscape Electrical
  Multimeter1 : powerlib/Measurements/Multimeter  PhasorSimulation=off  OutputType=Complex  sel=18  L=30  Gain=1  yselected={'Ib: DGU3/Resistance'};  PSBOutputType=1  PSBequivalent=0  AxesSetting=[0,0.1,-100,100]  Display=0  SavedBlockNames=-11
      settings: SourceProductName=Simscape Electrical
  Multimeter2 : powerlib/Measurements/Multimeter  PhasorSimulation=off  OutputType=Complex  sel=17  L=30  Gain=1  yselected={'Ib: DGU3/Capacitance'};  PSBOutputType=1  PSBequivalent=0  AxesSetting=[0,0.1,-100,100]  Display=0  SavedBlockNames=-11
      settings: SourceProductName=Simscape Electrical
  Multimeter3 : powerlib/Measurements/Multimeter  PhasorSimulation=off  OutputType=Complex  sel=27  L=30  Gain=1  yselected={'Isrc: DGU3/Controlled Current Source'};  PSBOutputType=1  PSBequivalent=0  AxesSetting=[0,0.1,-100,100]  Display=0  SavedBlockNames=-11
      settings: SourceProductName=Simscape Electrical
  Multimeter4 : powerlib/Measurements/Multimeter  PhasorSimulation=off  OutputType=Complex  sel=3  L=30  Gain=1  yselected={'Ub: DGU3/Capacitance'};  PSBOutputType=1  PSBequivalent=0  AxesSetting=[0,0.1,-100,100]  Display=0  SavedBlockNames=-11
      settings: SourceProductName=Simscape Electrical
  Primary  Voltage  Controller : Subsystem
  Product : Product
  Product1 : Product
  Resistance : powerlib/Elements/Series RLC Branch  LConnTagsString=__new0  RConnTagsString=__new0  BranchType=R  Resistance=DGU(3).Rt  Inductance=1e-3  SetiL0=off  InitialCurrent=0  Capacitance=1e-6  Setx0=off  InitialVoltage=0  Measurements=Branch current
      settings: SourceProductName=Simscape Electrical
  Scope{,1..4,6} (6 alike) : Scope
  Secondary  Consensus Layer : Subsystem  Commented=on
  Sum : Sum  Inputs=+|+
  Switch : Switch  Commented=on  Criteria=u2 ~= 0  Threshold=0.1
  Switching : Subsystem
  Voltage Measurement : powerlib/Measurements/Voltage Measurement  PhasorSimulation=off  OutputType=Complex  PSBequivalent=0
      settings: SourceProductName=Simscape Electrical
  ZIE Load : MATLAB Function  Commented=on  TreatAsAtomicUnit=on
  ZIE Load r>1 : MATLAB Function  Commented=on  TreatAsAtomicUnit=on
  ZIP Load : MATLAB Function  Commented=on  TreatAsAtomicUnit=on
  powergui1 : powerlib/powergui  Priority=1  Commented=on  SimulationMode=Continuous  SampleTime=50e-6  frequency=60  Iterations=50  frequencyindice=60  Pbase=100e6  ErrMax=1e-4  UnitsV=kV  UnitsW=MW  buscounter=0  FunctionMessages=off  echomessages=off  EnableUseOfTLC=off  CurrentSourceSwitches=off  DisableSnubberDevices=off  DisableRonSwitches=off  DisableVfSwitches=off  DisplayEquations=off  AutomaticDiscreteSolvers=off  SolverType=Tustin/Backward Euler (TBE)  Interpol=off  ExternalGateDelay=off  methode=off  Ts=100  x0status=blocks  SPID=on  SwTol=0  HookPort=off  NonlinearTolerance=1e-4  nMaxIteration=100  ContinueOnMaxIteration=off  RestoreLinks=warning  ResistiveCurrentMeasurement=off  Frange=[0:2:500]  Ylog=off  Xlog=on  ShowGrid=off  save=off  variable=ZData  structure=0  ZoomFFT=off  StartTime=0.0  cycles=1  DisplayStyle=1  fundamental=60  FreqAxis=off  MaxFrequency=1000  frequencyindicesteady=1  RmsSteady=1  display=off
      settings: SourceProductName=Simscape Electrical
  PCC3 : PMIOPort  Tag=PMCPort  Side=Left
  tag scope: Ic3=global, Il3=global, It3=global, V3=global, Vs3=global, Vt3=global
  wires:
  Multimeter/1 -> Scope/1, [Vs3]
  Multimeter2/1 -> Scope2/1, [Ic3]
  Voltage Measurement/1 -> Scope4/1, [Vt3]
  Multimeter1/1 -> Scope1/1, [It3]
  [SW_Buck_3n] -> IGBT1/1
  Multimeter3/1 -> Scope3/1, [Il3]
  [SW_Buck_3] -> IGBT/1
  Multimeter4/1 -> [V3]
  Mixed ZIP-ZIE Load/1(y) -> Controlled Current Source/1
  From4/1 -> Switch/2
  From3/1 -> Switch/1
  Constant/1 -> Switch/3
  [Vref3] -> Product1/1
  Product1/1 -> Sum/2
  Sum/1 -> Mixed ZIP-ZIE Load/1(u), Scope6/1
  [loadsNOT] -> Product1/2
  [loads] -> Product/2
  Memory/1 -> Product/1
  Product/1 -> Sum/1
  [V3] -> Memory/1
  Clock/1 -> Mixed ZIP-ZIE Load/2(time)
  connections:
  Ground1/LConn1 -- Voltage Measurement/LConn2
  IGBT1/RConn1 -- Controlled Current Source/RConn1 -- Capacitance/RConn1 -- Ground/LConn1 -- DC Voltage Source/LConn1 -- Diode1/LConn1
  IGBT/LConn1 -- Diode/RConn1 -- DC Voltage Source/RConn1
  Resistance/RConn1 -- Inductance/LConn1
  IGBT/RConn1 -- Resistance/LConn1 -- Voltage Measurement/LConn1 -- Diode1/RConn1 -- IGBT1/LConn1 -- Diode/LConn1
  Capacitance/LConn1 -- PCC3/RConn1 -- Controlled Current Source/LConn1 -- Inductance/RConn1

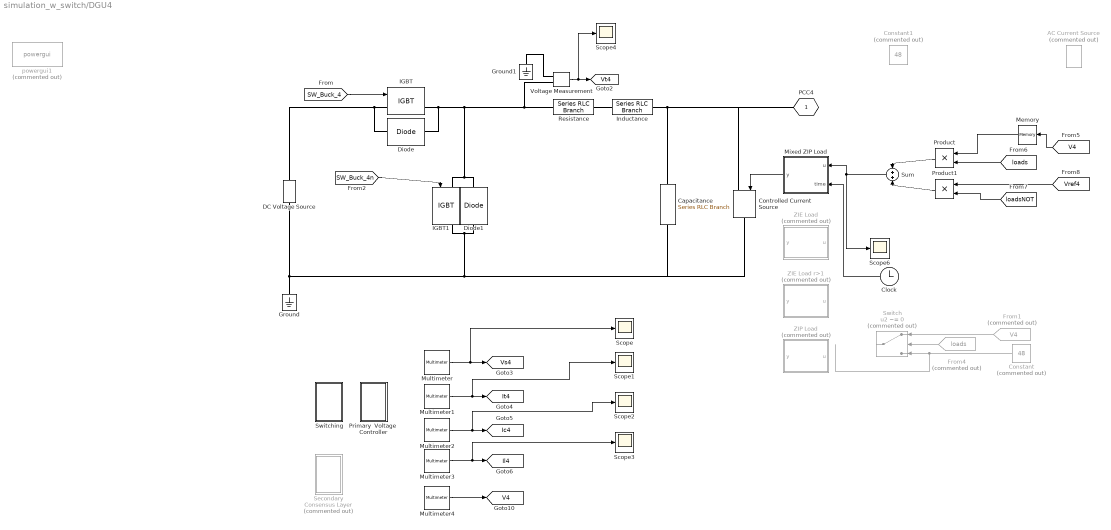
== system simulation_w_switch/DGU4 ==
  AC Current Source : powerlib/Electrical Sources/AC Current Source  Commented=on  Amplitude=13  Phase=90  Frequency=0  SampleTime=0  Measurements=Current
      settings: SourceProductName=Simscape Electrical  SourceProductBaseCode=PS
  Capacitance : powerlib/Elements/Series RLC Branch  LConnTagsString=__new0  RConnTagsString=__new0  BranchType=C  Resistance=1  Inductance=1.8e-3  SetiL0=off  InitialCurrent=0  Capacitance=DGU(4).Ct  Setx0=on  InitialVoltage=48  Measurements=Branch voltage and current
      settings: SourceProductName=Simscape Electrical
  Clock : Clock
  Constant : Constant  Commented=on  Value=48
  Constant1 : Constant  Commented=on  Value=48
  Controlled Current Source : powerlib/Electrical Sources/Controlled Current Source  Initialize=on  Source_Type=DC  Amplitude=Il_bar4  Phase=0  Frequency=0  Measurements=Current
      settings: SourceProductName=Simscape Electrical
  DC Voltage Source : powerlib/Electrical Sources/DC Voltage Source  Amplitude=Vs  Measurements=Voltage
      settings: SourceProductName=Simscape Electrical
  Diode : powerlib/Power Electronics/Diode  Ron=0.001  Lon=0  Vf=0.8  IC=0  UseSnubber=0  Rs=500  Cs=250e-9  Measurements=off
      settings: SourceProductName=Simscape Electrical
  Diode1 : powerlib/Power Electronics/Diode  Ron=0.001  Lon=0  Vf=0.8  IC=0  UseSnubber=0  Rs=500  Cs=250e-9  Measurements=off
      settings: SourceProductName=Simscape Electrical
  From1 : From  Commented=on  GotoTag=V4  TagVisibility=global
  From4 : From  Commented=on  GotoTag=loads  TagVisibility=global
  Ground : powerlib/Elements/Ground  LConnTagsString=a
      settings: SourceProductName=Simscape Electrical
  Ground1 : powerlib/Elements/Ground  LConnTagsString=a
      settings: SourceProductName=Simscape Electrical
  IGBT : powerlib/Power Electronics/IGBT  Ron=0.001  Lon=0  Vf=1  Tf=1e-6  Tt=2e-6  IC=0  Rs=1e5  Cs=inf  Measurements=on
      settings: SourceProductName=Simscape Electrical
  IGBT1 : powerlib/Power Electronics/IGBT  Ron=0.001  Lon=0  Vf=1  Tf=1e-6  Tt=2e-6  IC=0  Rs=1e5  Cs=inf  Measurements=on
      settings: SourceProductName=Simscape Electrical
  Inductance : powerlib/Elements/Series RLC Branch  LConnTagsString=__new0  RConnTagsString=__new0  BranchType=L  Resistance=1  Inductance=DGU(4).Lt  SetiL0=on  InitialCurrent=Il_bar4  Capacitance=1e-6  Setx0=off  InitialVoltage=0  Measurements=None
      settings: SourceProductName=Simscape Electrical
  Memory : Memory
  Mixed ZIP Load : MATLAB Function  TreatAsAtomicUnit=on
  Multimeter : powerlib/Measurements/Multimeter  PhasorSimulation=off  OutputType=Complex  sel=10  L=30  Gain=1  yselected={'Usrc: DGU4/DC Voltage Source'};  PSBOutputType=1  PSBequivalent=0  AxesSetting=[0,0.1,-100,100]  Display=0  SavedBlockNames=-11
      settings: SourceProductName=Simscape Electrical
  Multimeter1 : powerlib/Measurements/Multimeter  PhasorSimulation=off  OutputType=Complex  sel=20  L=30  Gain=1  yselected={'Ib: DGU4/Resistance'};  PSBOutputType=1  PSBequivalent=0  AxesSetting=[0,0.1,-100,100]  Display=0  SavedBlockNames=-11
      settings: SourceProductName=Simscape Electrical
  Multimeter2 : powerlib/Measurements/Multimeter  PhasorSimulation=off  OutputType=Complex  sel=19  L=30  Gain=1  yselected={'Ib: DGU4/Capacitance'};  PSBOutputType=1  PSBequivalent=0  AxesSetting=[0,0.1,-100,100]  Display=0  SavedBlockNames=-11
      settings: SourceProductName=Simscape Electrical
  Multimeter3 : powerlib/Measurements/Multimeter  PhasorSimulation=off  OutputType=Complex  sel=28  L=30  Gain=1  yselected={'Isrc: DGU4/Controlled Current Source'};  PSBOutputType=1  PSBequivalent=0  AxesSetting=[0,0.1,-100,100]  Display=0  SavedBlockNames=-11
      settings: SourceProductName=Simscape Electrical
  Multimeter4 : powerlib/Measurements/Multimeter  PhasorSimulation=off  OutputType=Complex  sel=4  L=30  Gain=1  yselected={'Ub: DGU4/Capacitance'};  PSBOutputType=1  PSBequivalent=0  AxesSetting=[0,0.1,-100,100]  Display=0  SavedBlockNames=-11
      settings: SourceProductName=Simscape Electrical
  Primary  Voltage  Controller : Subsystem
  Product : Product
  Product1 : Product
  Resistance : powerlib/Elements/Series RLC Branch  LConnTagsString=__new0  RConnTagsString=__new0  BranchType=R  Resistance=DGU(4).Rt  Inductance=1e-3  SetiL0=off  InitialCurrent=0  Capacitance=1e-6  Setx0=off  InitialVoltage=0  Measurements=Branch current
      settings: SourceProductName=Simscape Electrical
  Scope{,1..4,6} (6 alike) : Scope
  Secondary Consensus Layer : Subsystem  Commented=on
  Sum : Sum  Inputs=+|+
  Switch : Switch  Commented=on  Criteria=u2 ~= 0  Threshold=0.1
  Switching : Subsystem
  Voltage Measurement : powerlib/Measurements/Voltage Measurement  PhasorSimulation=off  OutputType=Complex  PSBequivalent=0
      settings: SourceProductName=Simscape Electrical
  ZIE Load : MATLAB Function  Commented=on  TreatAsAtomicUnit=on
  ZIE Load r>1 : MATLAB Function  Commented=on  TreatAsAtomicUnit=on
  ZIP Load : MATLAB Function  Commented=on  TreatAsAtomicUnit=on
  powergui1 : powerlib/powergui  Priority=1  Commented=on  SimulationMode=Continuous  SampleTime=50e-6  frequency=60  Iterations=50  frequencyindice=60  Pbase=100e6  ErrMax=1e-4  UnitsV=kV  UnitsW=MW  buscounter=0  FunctionMessages=off  echomessages=off  EnableUseOfTLC=off  CurrentSourceSwitches=off  DisableSnubberDevices=off  DisableRonSwitches=off  DisableVfSwitches=off  DisplayEquations=off  AutomaticDiscreteSolvers=off  SolverType=Tustin/Backward Euler (TBE)  Interpol=off  ExternalGateDelay=off  methode=off  Ts=100  x0status=blocks  SPID=on  SwTol=0  HookPort=off  NonlinearTolerance=1e-4  nMaxIteration=100  ContinueOnMaxIteration=off  RestoreLinks=warning  ResistiveCurrentMeasurement=off  Frange=[0:2:500]  Ylog=off  Xlog=on  ShowGrid=off  save=off  variable=ZData  structure=0  ZoomFFT=off  StartTime=0.0  cycles=1  DisplayStyle=1  fundamental=60  FreqAxis=off  MaxFrequency=1000  frequencyindicesteady=1  RmsSteady=1  display=off
      settings: SourceProductName=Simscape Electrical
  PCC4 : PMIOPort  Tag=PMCPort  Side=Left
  tag scope: Ic4=global, Il4=global, It4=global, V4=global, Vs4=global, Vt4=global
  wires:
  Multimeter/1 -> Scope/1, [Vs4]
  Multimeter2/1 -> Scope2/1, [Ic4]
  Voltage Measurement/1 -> Scope4/1, [Vt4]
  Multimeter1/1 -> Scope1/1, [It4]
  [SW_Buck_4n] -> IGBT1/1
  Multimeter3/1 -> Scope3/1, [Il4]
  [SW_Buck_4] -> IGBT/1
  Multimeter4/1 -> [V4]
  Mixed ZIP Load/1(y) -> Controlled Current Source/1
  From4/1 -> Switch/2
  From1/1 -> Switch/1
  Constant/1 -> Switch/3
  [Vref4] -> Product1/1
  Product1/1 -> Sum/2
  Sum/1 -> Mixed ZIP Load/1(u), Scope6/1
  [loadsNOT] -> Product1/2
  [loads] -> Product/2
  Memory/1 -> Product/1
  Product/1 -> Sum/1
  [V4] -> Memory/1
  Clock/1 -> Mixed ZIP Load/2(time)
  connections:
  Ground1/LConn1 -- Voltage Measurement/LConn2
  IGBT1/RConn1 -- Controlled Current Source/RConn1 -- Capacitance/RConn1 -- Ground/LConn1 -- DC Voltage Source/LConn1 -- Diode1/LConn1
  IGBT/LConn1 -- Diode/RConn1 -- DC Voltage Source/RConn1
  Resistance/RConn1 -- Inductance/LConn1
  IGBT/RConn1 -- Resistance/LConn1 -- Voltage Measurement/LConn1 -- Diode1/RConn1 -- IGBT1/LConn1 -- Diode/LConn1
  Capacitance/LConn1 -- PCC4/RConn1 -- Controlled Current Source/LConn1 -- Inductance/RConn1
